simulink library "rocket_vertical_flight_library"  (R2014a)
settings: Solver=ode45  StartTime=0.0  StopTime=10.0  RelTol=1e-3
settings Model: Creator=scorpii  LastModifiedBy=scorpii

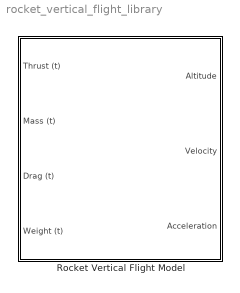
== system rocket_vertical_flight_library ==
  Rocket Vertical Flight Model : Subsystem

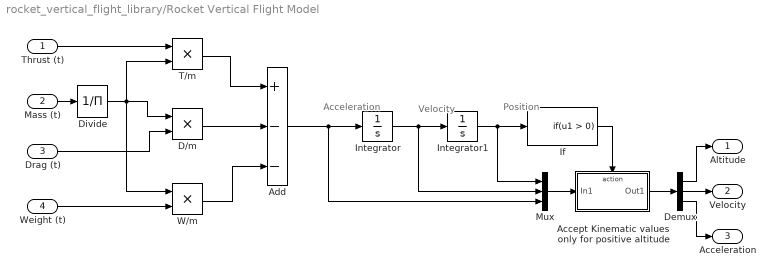
== system rocket_vertical_flight_library/Rocket Vertical Flight Model ==
  note: Acceleration
  note: Position
  note: Velocity
  Thrust (t) : Inport
  Mass (t) : Inport  Port=2
  Drag (t) : Inport  Port=3
  Weight (t) : Inport  Port=4
  Accept Kinematic values only for positive altitude : Subsystem  TreatAsAtomicUnit=on
  Add : Sum  Inputs=+--
  D/m : Product
  Demux : Demux  Outputs=3
  Divide : Product  Inputs=/
  If : If  ShowElse=off
  Integrator : Integrator
  Integrator1 : Integrator
  Mux : Mux  Inputs=3
  T/m : Product
  W/m : Product
  Altitude : Outport
  Velocity : Outport  Port=2
  Acceleration : Outport  Port=3
  wires:
  Divide/1 -> W/m/1, D/m/1, T/m/2
  W/m/1 -> Add/3
  D/m/1 -> Add/2
  T/m/1 -> Add/1
  Add/1 -> Mux/3, Integrator/1
  Integrator/1 -> Integrator1/1, Mux/2
  Integrator1/1 -> Mux/1, If/1
  Drag (t)/1 -> D/m/2
  Mass (t)/1 -> Divide/1
  Weight (t)/1 -> W/m/2
  Thrust (t)/1 -> T/m/1
  If/1 -> Accept Kinematic values only for positive altitude/Action
  Mux/1 -> Accept Kinematic values only for positive altitude/1(In1)
  Accept Kinematic values only for positive altitude/1(Out1) -> Demux/1
  Demux/1 -> Altitude/1
  Demux/2 -> Velocity/1
  Demux/3 -> Acceleration/1

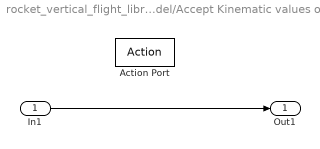
== system rocket_vertical_flight_library/Rocket Vertical Flight Model/Accept Kinematic values only for positive altitude ==
  In1 : Inport
  Action Port : ActionPort  ActionType=then
  Out1 : Outport
  wires:
  In1/1 -> Out1/1
